simulink model "LySim"  (R2022a)
settings: Solver=ode113  StartTime=0.0  StopTime=100  RelTol=1e-4
values from neighbouring files (symbols this model uses):
  x_goal = pos(i,1)    [DataProcess.m]
  y_goal = pos(i,2)    [DataProcess.m]
settings Model: Creator=Xu  LastModifiedBy=Xu
settings SolverCC: MaxConsecutiveMinStep=10  ShapePreserveControl=EnableAll  ODENIntegrationMethod=ode1be

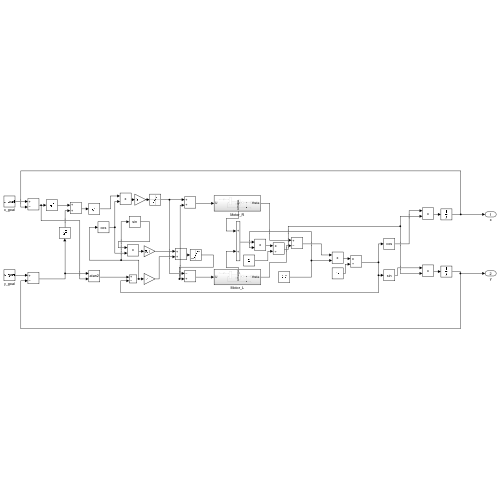
[thumbnail: Simulink's stored preview of the top-level diagram]
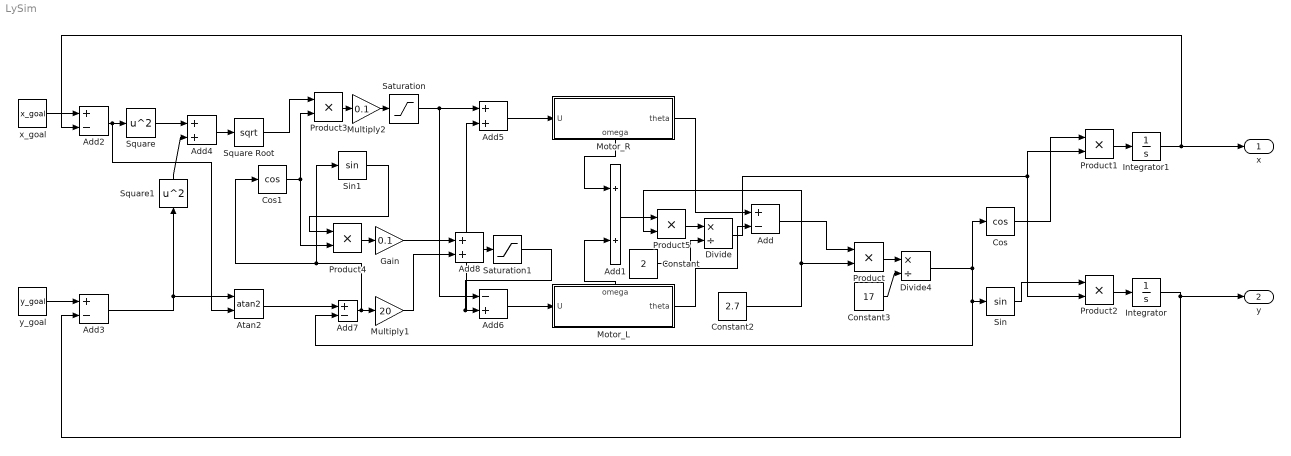
== system LySim ==
  Add{,2..3,7} (4 alike) : Sum  Inputs=+-
  Add{1,4..5,8} (4 alike) : Sum
  Add6 : Sum  Inputs=-+
  Atan2 : Trigonometry  Operator=atan2
  Constant : Constant  Value=2
  Constant2 : Constant  Value=2.7
  Constant3 : Constant  Value=17
  Cos : Trigonometry  Operator=cos
  Cos1 : Trigonometry  Operator=cos
  Divide : Product  Inputs=*/
  Divide4 : Product  Inputs=*/
  Gain : Gain  Gain=0.1
  Integrator : Integrator
  Integrator1 : Integrator
  Motor_L : Subsystem
      settings: PortSchema="{\"entries\":[{\"content\":{\"sides\":[{\"content\":{\"connectorIds\":[\"In1\"]},\"type\":\"ConnectorPlacement.EquallySpacedRectSide\",\"uuid\":\"8a442169-6c77-460c-a00b-bb58efc2ee11\"},{\"content\":{\"connectorIds\":[\"Out1\"],\"side\":\"RIGHT\"},\"type\":\"ConnectorPlacement.EquallySpacedRectSide\",\"uuid\":\"37accc6a-9d02-4149-a232-0c0e22d63e0d\"},{\"content\":{\"connectorIds\":[\"Out2\"],\"side\":\"TOP\"},\"type\":\"ConnectorPlacement.EquallySpacedRectSide\",\"uuid\":\"f525baf1-e508-41af-b7c6-1372207e0b7e\"},{\"content\":{\"connectorIds\":[],\"side\":\"BOTTOM\"},\"type\":\"ConnectorPlacement.EquallySpacedRectSide\",\"uuid\":\"065ecf0b-8beb-4240-a5e1-1e7a5625764c\"}]},\"type\":\"ConnectorPlacement.EquallySpacedConnector\",\"uuid\":\"0a4b1493-27e4-4c9d-b9fc-2ddd89bc15b2\"}],\"packageUris\":[\"http://schema.mathworks.com/mf0/Connector/R2020b\"],\"version\":\"1.0\"}"
  Motor_R : Subsystem
      settings: PortSchema="{\"entries\":[{\"content\":{\"sides\":[{\"content\":{\"connectorIds\":[\"In1\"]},\"type\":\"ConnectorPlacement.EquallySpacedRectSide\",\"uuid\":\"8a442169-6c77-460c-a00b-bb58efc2ee11\"},{\"content\":{\"connectorIds\":[\"Out1\"],\"side\":\"RIGHT\"},\"type\":\"ConnectorPlacement.EquallySpacedRectSide\",\"uuid\":\"37accc6a-9d02-4149-a232-0c0e22d63e0d\"},{\"content\":{\"connectorIds\":[],\"side\":\"TOP\"},\"type\":\"ConnectorPlacement.EquallySpacedRectSide\",\"uuid\":\"f525baf1-e508-41af-b7c6-1372207e0b7e\"},{\"content\":{\"connectorIds\":[\"Out2\"],\"side\":\"BOTTOM\"},\"type\":\"ConnectorPlacement.EquallySpacedRectSide\",\"uuid\":\"c227137f-2e52-455e-aa84-1df2c1c3622a\"}]},\"type\":\"ConnectorPlacement.EquallySpacedConnector\",\"uuid\":\"0a4b1493-27e4-4c9d-b9fc-2ddd89bc15b2\"}],\"packageUris\":[\"http://schema.mathworks.com/mf0/Connector/R2020b\"],\"version\":\"1.0\"}"
  Multiply1 : Gain  Gain=20
  Multiply2 : Gain  Gain=0.1
  Product{,1..5} (6 alike) : Product
  Saturation : Saturate  UpperLimit=3  LowerLimit=-3
  Saturation1 : Saturate  UpperLimit=4  LowerLimit=-4
  Sin : Trigonometry
  Sin1 : Trigonometry
  Square : Math  Operator=square
  Square Root : Sqrt
  Square1 : Math  Operator=square
  x_goal : Constant  Value=x_goal
  y_goal : Constant  Value=y_goal
  x : Outport
  y : Outport  Port=2
  wires:
  Divide/1 -> Product2/2, Product1/2
  Sin/1 -> Product2/1
  Motor_R/1(theta) -> Add/1
  Motor_L/1(theta) -> Add/2
  Add/1 -> Product/1
  Constant2/1 -> Product5/2, Product/2
  Product/1 -> Divide4/1
  Constant3/1 -> Divide4/2
  Motor_R/2(omega) -> Add1/1
  Motor_L/2(omega) -> Add1/2
  Add1/1 -> Product5/1
  Constant/1 -> Divide/2
  Cos/1 -> Product1/1
  Divide4/1 -> Cos/1, Add7/2, Sin/1
  Product1/1 -> Integrator1/1
  Product2/1 -> Integrator/1
  x_goal/1 -> Add2/1
  y_goal/1 -> Add3/1
  Add3/1 -> Atan2/1, Square1/1
  Square1/1 -> Add4/2
  Square/1 -> Add4/1
  Add4/1 -> Square Root/1
  Saturation1/1 -> Add6/2, Add5/2
  Add7/1 -> Sin1/1, Cos1/1, Multiply1/1
  Atan2/1 -> Add7/1
  Product3/1 -> Multiply2/1
  Add6/1 -> Motor_L/1(U)
  Add5/1 -> Motor_R/1(U)
  Saturation/1 -> Add6/1, Add5/1
  Multiply1/1 -> Add8/2
  Multiply2/1 -> Saturation/1
  Sin1/1 -> Product4/1
  Add8/1 -> Saturation1/1
  Gain/1 -> Add8/1
  Add2/1 -> Atan2/2, Square/1
  Integrator/1 -> Add3/2, y/1
  Integrator1/1 -> x/1, Add2/2
  Square Root/1 -> Product3/1
  Cos1/1 -> Product3/2, Product4/2
  Product4/1 -> Gain/1
  Product5/1 -> Divide/1

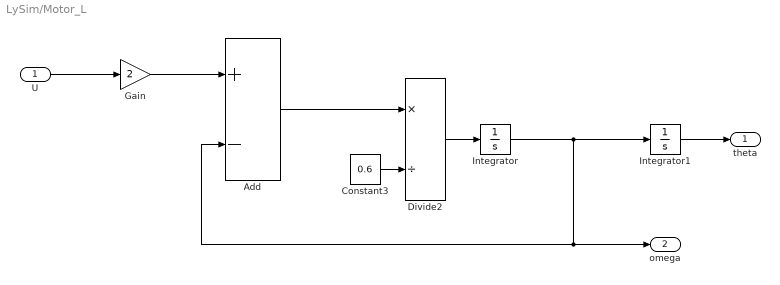
== system LySim/Motor_L ==
  U : Inport
  Add : Sum  Inputs=+-
  Constant3 : Constant  Value=0.6
  Divide2 : Product  Inputs=*/
  Gain : Gain  Gain=2
  Integrator : Integrator
  Integrator1 : Integrator
  theta : Outport
  omega : Outport  Port=2
  wires:
  Integrator1/1 -> theta/1
  Divide2/1 -> Integrator/1
  Integrator/1 -> omega/1, Add/2, Integrator1/1
  Add/1 -> Divide2/1
  U/1 -> Gain/1
  Constant3/1 -> Divide2/2
  Gain/1 -> Add/1

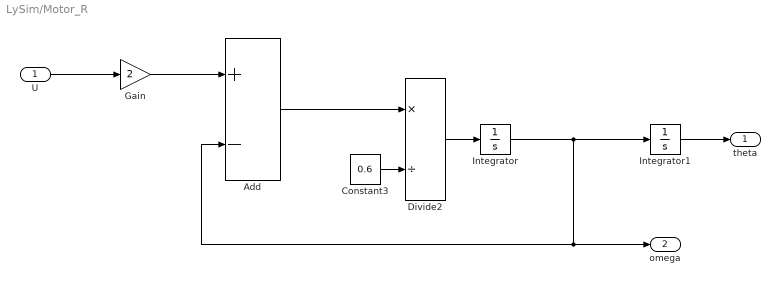
== system LySim/Motor_R ==
  U : Inport
  Add : Sum  Inputs=+-
  Constant3 : Constant  Value=0.6
  Divide2 : Product  Inputs=*/
  Gain : Gain  Gain=2
  Integrator : Integrator
  Integrator1 : Integrator
  theta : Outport
  omega : Outport  Port=2
  wires:
  Integrator1/1 -> theta/1
  Divide2/1 -> Integrator/1
  Integrator/1 -> omega/1, Add/2, Integrator1/1
  Add/1 -> Divide2/1
  U/1 -> Gain/1
  Constant3/1 -> Divide2/2
  Gain/1 -> Add/1
